simulink model "chap9_6sim"  (Simulink 5.0)
settings: Solver=ode45  StartTime=0.0  StopTime=10  RelTol=1e-3
settings Model: LastModifiedBy=Administrator

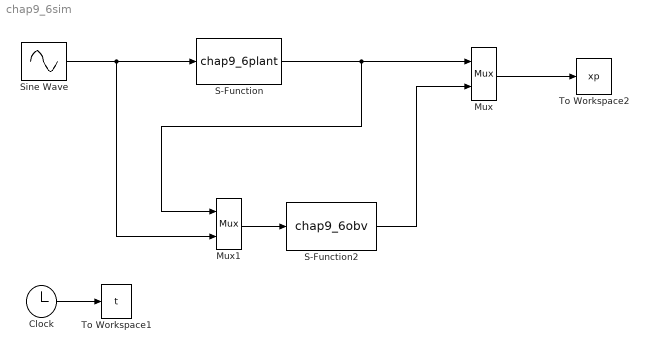
== system chap9_6sim ==
  Clock : Clock
      settings: Decimation=10
  Mux : Mux  Inputs=2
  Mux1 : Mux  Inputs=2
  S-Function : S-Function  FunctionName=chap9_6plant
  S-Function2 : S-Function  FunctionName=chap9_6obv
  Sine Wave : Sin  Frequency=2*pi  SampleTime=0
  To Workspace1 : ToWorkspace  VariableName=t  SampleTime=-1  SaveFormat=Array
  To Workspace2 : ToWorkspace  VariableName=xp  SampleTime=-1  SaveFormat=Array
  wires:
  Sine Wave/1 -> S-Function/1, Mux1/2
  S-Function/1 -> Mux/1, Mux1/1
  Clock/1 -> To Workspace1/1
  Mux1/1 -> S-Function2/1
  Mux/1 -> To Workspace2/1
  S-Function2/1 -> Mux/2
